simulink model "t_wit_sim"  (R2014a)
settings: Solver=ode45  StartTime=0.0  StopTime=10.0  RelTol=1e-3
values from neighbouring files (symbols this model uses):
  A_r = [0 1;0 0]    [T_WIT.m]    (also in t_wit_w_motor_model.m)
  A_t = zeros(4,4)    [T_WIT.m]    (also in t_wit_w_motor_model.m)
  B_r = [0;6/((9*Mr+Mp)*R*D)]    [T_WIT.m]    (also in t_wit_w_motor_model.m)
  B_t = zeros(4,1)    [T_WIT.m]    (also in t_wit_w_motor_model.m)
  C_r = eye(2)    [T_WIT.m]    (also in t_wit_w_motor_model.m)
  C_t = eye(4)    [T_WIT.m]    (also in t_wit_w_motor_model.m)
  D_r = zeros(2,1)    [T_WIT.m]    (also in t_wit_w_motor_model.m)
  D_t = zeros(4,1)    [T_WIT.m]    (also in t_wit_w_motor_model.m)
  K1 = lqr(A_t,B_t,Q,R)    [T_WIT.m]    (also in t_wit_w_motor_model.m = place(A_t,B_t,p1))
  K2 = place(A_r,B_r,p2)    [T_WIT.m]    (also in t_wit_w_motor_model.m)
  Psi_dot_in = 0*(pi/180)    (= 0)    [T_WIT.m]    (also in t_wit_w_motor_model.m)
  Theta_d = 5*(pi/180)    (= 0.0872664625997)    [T_WIT.m]    (also in t_wit_w_motor_model.m = 0.523598775598)
  V_in = 0.00    (= 0)    [T_WIT.m]    (also in t_wit_w_motor_model.m)
settings Model: CovSFcnEnable=on  Creator=jz4hf  LastModifiedBy=jeson_000
settings OptimizationCC: SimCompilerOptimization=off
settings DebuggingCC: MergeDetectMultiDrivingBlocksExec=error  SolverPrmCheckMsg=none  FrameProcessingCompatibilityMsg=error
settings RTWCC: RTWCompilerOptimization=off

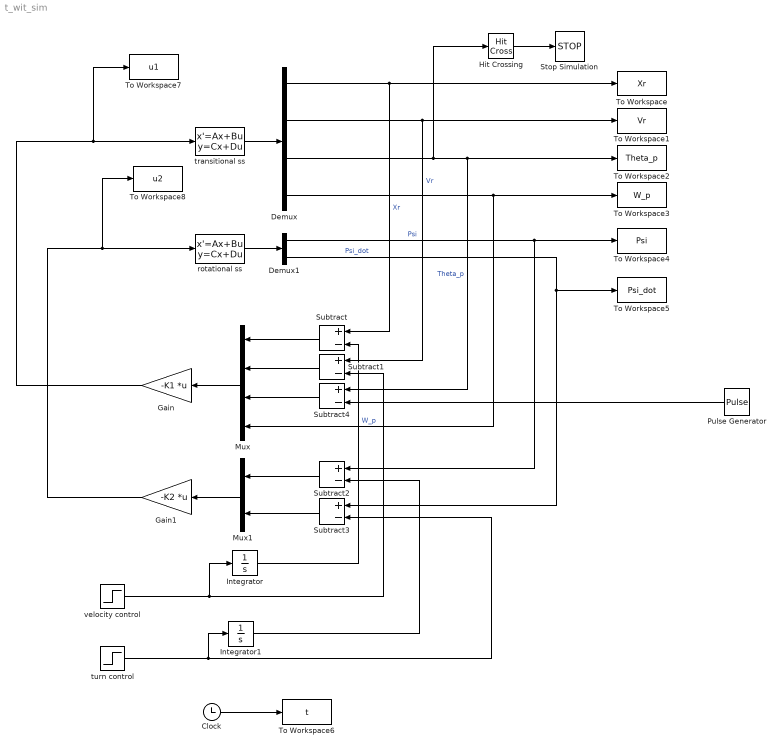
== system t_wit_sim ==
  Clock : Clock
  Demux : Demux
  Demux1 : Demux  Outputs=2
  Gain : Gain  Gain=-K1  Multiplication=Matrix(K*u)
  Gain1 : Gain  Gain=-K2  Multiplication=Matrix(K*u)
  Hit Crossing : HitCross  HitCrossingOffset=-pi/2
  Integrator : Integrator
  Integrator1 : Integrator
  Mux : Mux
  Mux1 : Mux  Inputs=2
  Pulse Generator : DiscretePulseGenerator  PulseType=Time based  Amplitude=Theta_d  Period=20  PulseWidth=0.5
  Stop Simulation : Stop
  Subtract{,1..4} (5 alike) : Sum  Inputs=+-
  To Workspace : ToWorkspace  VariableName=Xr  SampleTime=-1
  To Workspace1 : ToWorkspace  VariableName=Vr  SampleTime=-1
  To Workspace2 : ToWorkspace  VariableName=Theta_p  SampleTime=-1
  To Workspace3 : ToWorkspace  VariableName=W_p  SampleTime=-1
  To Workspace4 : ToWorkspace  VariableName=Psi  SampleTime=-1
  To Workspace5 : ToWorkspace  VariableName=Psi_dot  SampleTime=-1
  To Workspace6 : ToWorkspace  VariableName=t  SampleTime=-1
  To Workspace7 : ToWorkspace  VariableName=u1  SampleTime=-1
  To Workspace8 : ToWorkspace  VariableName=u2  SampleTime=-1
  rotational ss : StateSpace  A=A_r  B=B_r  C=C_r  D=D_r  X0=0
  transitional ss : StateSpace  A=A_t  B=B_t  C=C_t  D=D_t  X0=0
  turn control : Step  After=Psi_dot_in  SampleTime=0
  velocity control : Step  After=V_in  SampleTime=0
  wires:
  transitional ss/1 -> Demux/1
  Demux/1 -> Subtract/1, To Workspace/1  "Xr"
  Demux/2 -> Subtract1/1, To Workspace1/1  "Vr"
  Demux/3 -> Hit Crossing/1, Subtract4/1, To Workspace2/1  "Theta_p"
  Demux/4 -> Mux/4, To Workspace3/1  "W_p"
  Demux1/1 -> Subtract2/1, To Workspace4/1  "Psi"
  Demux1/2 -> Subtract3/1, To Workspace5/1  "Psi_dot"
  Mux/1 -> Gain/1
  Mux1/1 -> Gain1/1
  Gain/1 -> To Workspace7/1, transitional ss/1
  Gain1/1 -> To Workspace8/1, rotational ss/1
  velocity control/1 -> Integrator/1, Subtract1/2
  Integrator/1 -> Subtract/2
  Subtract/1 -> Mux/1
  Subtract1/1 -> Mux/2
  Pulse Generator/1 -> Subtract4/2
  Subtract4/1 -> Mux/3
  turn control/1 -> Integrator1/1, Subtract3/2
  Integrator1/1 -> Subtract2/2
  Subtract2/1 -> Mux1/1
  Subtract3/1 -> Mux1/2
  Clock/1 -> To Workspace6/1
  rotational ss/1 -> Demux1/1
  Hit Crossing/1 -> Stop Simulation/1
